simulink model "traffic_light_stateflow"  (R2024b)
settings: Solver=ode3  StartTime=0.0  StopTime=50.0  FixedStep=1  RelTol=1e-3
settings Model: Creator=balaj  LastModifiedBy=balaj

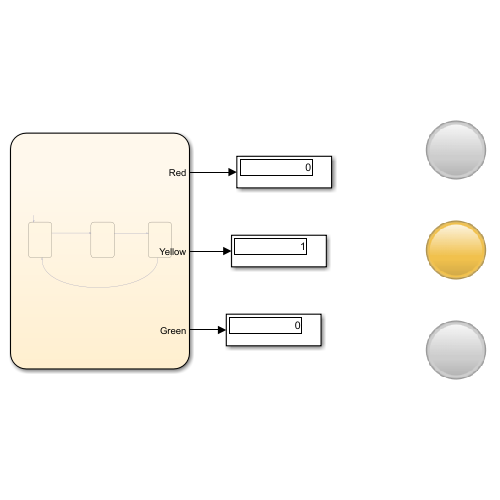
[thumbnail: Simulink's stored preview of the top-level diagram]
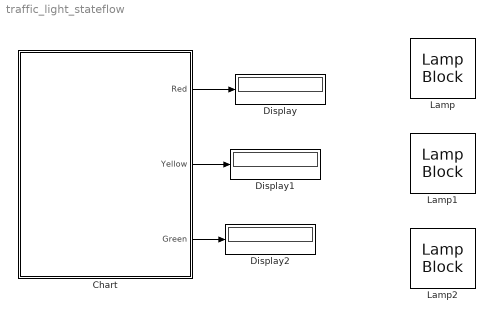
== system traffic_light_stateflow ==
  Chart : Stateflow chart  TreatAsAtomicUnit=on
  Display : Display
  Display1 : Display
  Display2 : Display
  Lamp : LampBlock  LabelPosition=Hide
  Lamp1 : LampBlock  LabelPosition=Hide
  Lamp2 : LampBlock  LabelPosition=Hide
  wires:
  Chart/1(Red) -> Display/1
  Chart/2(Yellow) -> Display1/1
  Chart/3(Green) -> Display2/1

== stateflow chart traffic_light_stateflow/Chart ==
  state PREPARETOGO
    entry:
    Red=0;
    Yellow=1;
    Green=0;
  state GO
    entry:
    Red=0;
    Yellow=0;
    Green=1;
  state STOP
    entry:
    Red=1;
    Yellow=0;
    Green=0;
  (default) -> STOP
  STOP -> PREPARETOGO : after(3,sec)
  PREPARETOGO -> GO : after(5,sec)
  GO -> STOP : after(7,sec)
  data: Red output; Yellow output; Green output
